simulink model "util_gravity_gradient_hrn"  (R2014b)
settings: Solver=VariableStepDiscrete  StartTime=0.0  StopTime=10.0  RelTol=1e-3
undefined symbols (not defined in the file or in its folder): csu_srp_solar_radiation_model_lib, gravity_gradient_torque, grv_mu_moon, I_sc, pos_m2sc_I, pos_sc2moon_body, q_body_from_mci
libraries: util_common_lib x9, util_info_lib x4, util_quat_lib x2
settings Model: Creator=Bryan Chan  LastModifiedBy=mstewart
settings DebuggingCC: UnderspecifiedInitializationDetection=Classic  MergeDetectMultiDrivingBlocksExec=none  SolverPrmCheckMsg=none  StateNameClashWarn=warning

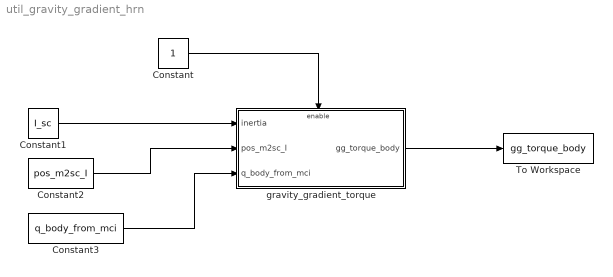
== system util_gravity_gradient_hrn ==
  Constant : Constant
  Constant1 : Constant  Value=I_sc
  Constant2 : Constant  Value=pos_m2sc_I
  Constant3 : Constant  Value=q_body_from_mci
  To Workspace : ToWorkspace  VariableName=gg_torque_body  SaveFormat=Timeseries  SampleTime=-1
  gravity_gradient_torque : Subsystem  AncestorBlock=csu_srp_solar_radiation_model_lib/gravity_gradient_torque
  wires:
  Constant/1 -> gravity_gradient_torque/Enable
  Constant1/1 -> gravity_gradient_torque/1(inertia)
  gravity_gradient_torque/1(gg_torque_body) -> To Workspace/1
  Constant2/1 -> gravity_gradient_torque/2(pos_m2sc_I)
  Constant3/1 -> gravity_gradient_torque/3(q_body_from_mci)

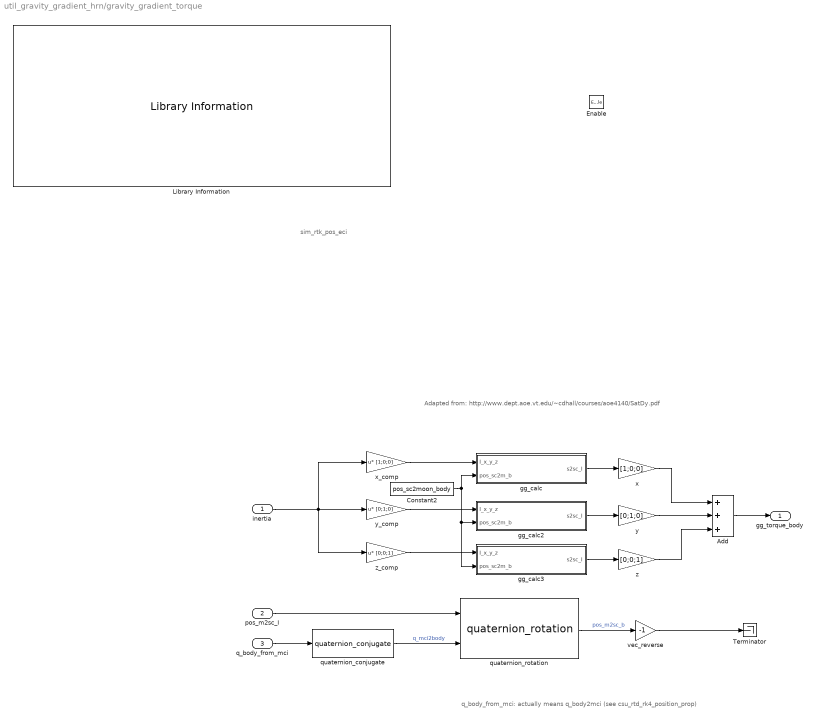
== system util_gravity_gradient_hrn/gravity_gradient_torque ==
  note: sim_rtk_pos_eci
  note: Adapted from: http://www.dept.aoe.vt.edu/~cdhall/courses/aoe4140/SatDy.pdf
  note: q_body_from_mci: actually means q_body2mci (see csu_rtd_rk4_position_prop)
  inertia : Inport
  pos_m2sc_I : Inport  Port=2
  q_body_from_mci : Inport  Port=3
  Enable : EnablePort
  Add : Sum  Inputs=+++
  Constant2 : Constant  Value=pos_sc2moon_body
  Library Information : util_info_lib/Library Information  owner='NONE'
  Terminator : Terminator
  gg_calc : Subsystem
  gg_calc2 : Subsystem
  gg_calc3 : Subsystem
  quaternion_conjugate : util_quat_lib/quaternion_conjugate  SystemSampleTime=-1
  quaternion_rotation : util_quat_lib/quaternion_rotation  SystemSampleTime=-1
  vec_reverse : Gain  Gain=-1
  x : Gain  Gain=[1;0;0]
  x_comp : Gain  Gain=[1;0;0]  Multiplication=Matrix(u*K)
  y : Gain  Gain=[0;1;0]
  y_comp : Gain  Gain=[0;1;0]  Multiplication=Matrix(u*K)
  z : Gain  Gain=[0;0;1]
  z_comp : Gain  Gain=[0;0;1]  Multiplication=Matrix(u*K)
  gg_torque_body : Outport
  wires:
  gg_calc3/1(s2sc_I) -> z/1
  gg_calc2/1(s2sc_I) -> y/1
  gg_calc/1(s2sc_I) -> x/1
  Constant2/1 -> gg_calc/2(pos_sc2m_b), gg_calc3/2(pos_sc2m_b), gg_calc2/2(pos_sc2m_b)
  z_comp/1 -> gg_calc3/1(I_x_y_z)
  y_comp/1 -> gg_calc2/1(I_x_y_z)
  x_comp/1 -> gg_calc/1(I_x_y_z)
  Add/1 -> gg_torque_body/1
  inertia/1 -> y_comp/1, z_comp/1, x_comp/1
  vec_reverse/1 -> Terminator/1
  quaternion_rotation/1 -> vec_reverse/1  "pos_m2sc_b"
  quaternion_conjugate/1 -> quaternion_rotation/2  "q_mci2body"
  q_body_from_mci/1 -> quaternion_conjugate/1
  pos_m2sc_I/1 -> quaternion_rotation/1
  x/1 -> Add/1
  y/1 -> Add/2
  z/1 -> Add/3

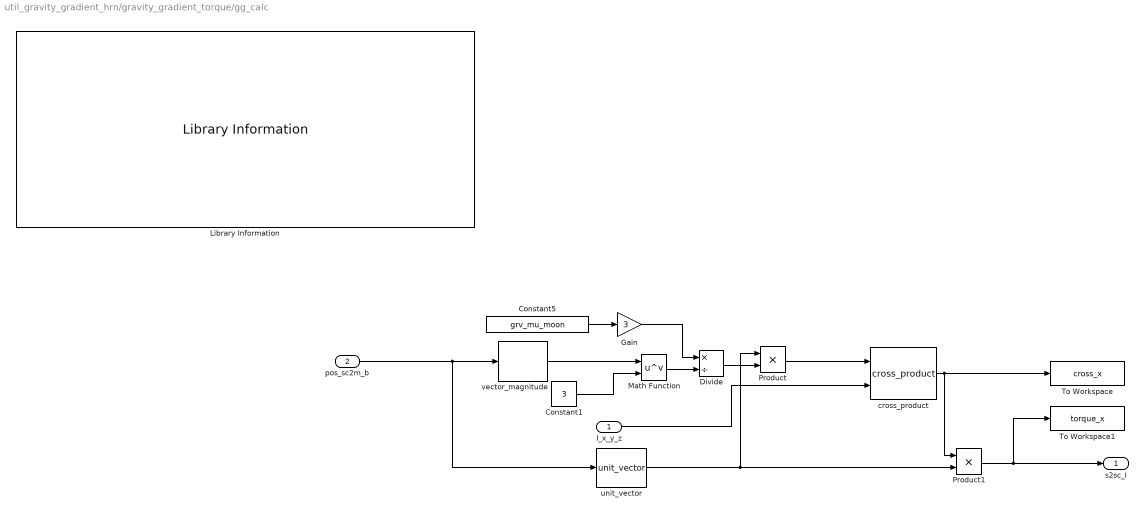
== system util_gravity_gradient_hrn/gravity_gradient_torque/gg_calc ==
  I_x_y_z : Inport
  pos_sc2m_b : Inport  Port=2
  Constant1 : Constant  Value=3
  Constant5 : Constant  Value=grv_mu_moon
  Divide : Product  Inputs=*/
  Gain : Gain  Gain=3
  Library Information : util_info_lib/Library Information  owner='NONE'
  Math Function : Math  Operator=pow  SaturateOnIntegerOverflow=on
  Product : Product
  Product1 : Product
  To Workspace : ToWorkspace  VariableName=cross_x  SaveFormat=Timeseries  SampleTime=-1
  To Workspace1 : ToWorkspace  VariableName=torque_x  SaveFormat=Timeseries  SampleTime=-1
  cross_product : util_common_lib/cross_product  SystemSampleTime=-1
  unit_vector : util_common_lib/unit_vector  SystemSampleTime=-1
  vector_magnitude : util_common_lib/vector_magnitude  SystemSampleTime=-1
  s2sc_I : Outport
  wires:
  pos_sc2m_b/1 -> vector_magnitude/1, unit_vector/1
  unit_vector/1 -> Product1/2, Product/1
  Math Function/1 -> Divide/2
  Gain/1 -> Divide/1
  Constant5/1 -> Gain/1
  Constant1/1 -> Math Function/2
  vector_magnitude/1 -> Math Function/1
  I_x_y_z/1 -> cross_product/2
  cross_product/1 -> Product1/1, To Workspace/1
  Divide/1 -> Product/2
  Product/1 -> cross_product/1
  Product1/1 -> To Workspace1/1, s2sc_I/1

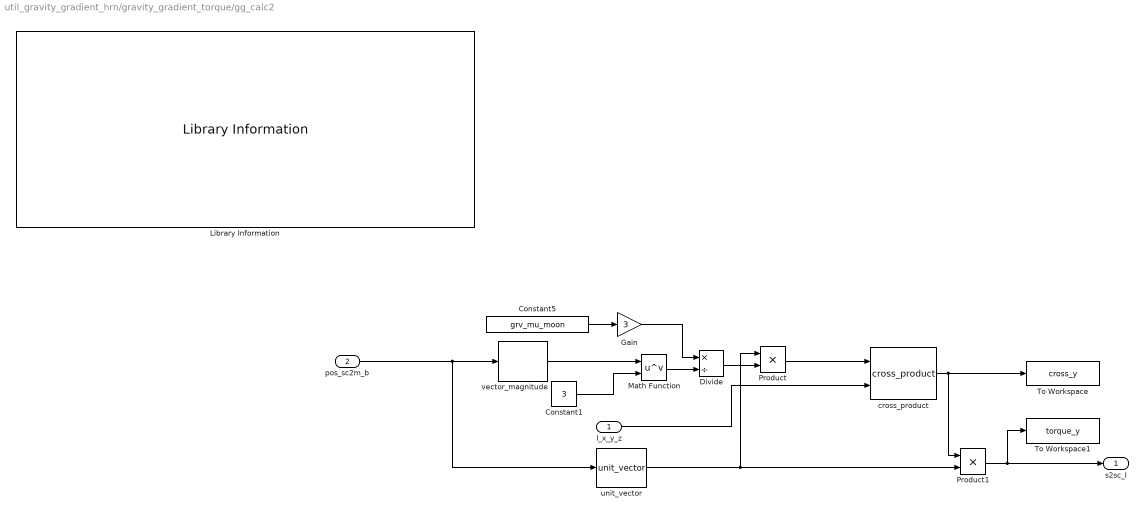
== system util_gravity_gradient_hrn/gravity_gradient_torque/gg_calc2 ==
  I_x_y_z : Inport
  pos_sc2m_b : Inport  Port=2
  Constant1 : Constant  Value=3
  Constant5 : Constant  Value=grv_mu_moon
  Divide : Product  Inputs=*/
  Gain : Gain  Gain=3
  Library Information : util_info_lib/Library Information  owner='NONE'
  Math Function : Math  Operator=pow  SaturateOnIntegerOverflow=on
  Product : Product
  Product1 : Product
  To Workspace : ToWorkspace  VariableName=cross_y  SaveFormat=Timeseries  SampleTime=-1
  To Workspace1 : ToWorkspace  VariableName=torque_y  SaveFormat=Timeseries  SampleTime=-1
  cross_product : util_common_lib/cross_product  SystemSampleTime=-1
  unit_vector : util_common_lib/unit_vector  SystemSampleTime=-1
  vector_magnitude : util_common_lib/vector_magnitude  SystemSampleTime=-1
  s2sc_I : Outport
  wires:
  Product1/1 -> To Workspace1/1, s2sc_I/1
  Product/1 -> cross_product/1
  Divide/1 -> Product/2
  cross_product/1 -> To Workspace/1, Product1/1
  I_x_y_z/1 -> cross_product/2
  vector_magnitude/1 -> Math Function/1
  Constant1/1 -> Math Function/2
  Constant5/1 -> Gain/1
  Gain/1 -> Divide/1
  Math Function/1 -> Divide/2
  unit_vector/1 -> Product1/2, Product/1
  pos_sc2m_b/1 -> unit_vector/1, vector_magnitude/1

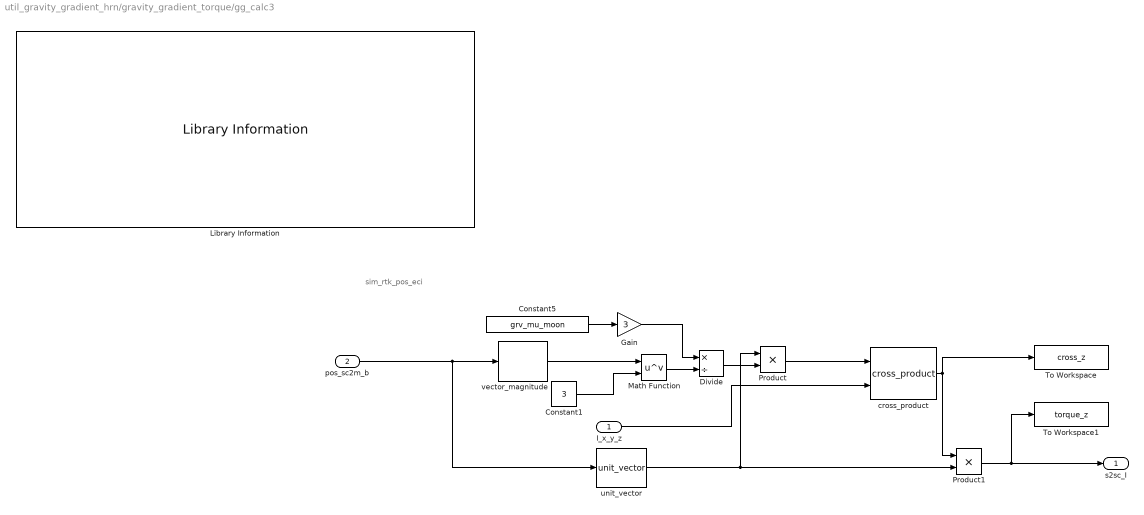
== system util_gravity_gradient_hrn/gravity_gradient_torque/gg_calc3 ==
  note: sim_rtk_pos_eci
  I_x_y_z : Inport
  pos_sc2m_b : Inport  Port=2
  Constant1 : Constant  Value=3
  Constant5 : Constant  Value=grv_mu_moon
  Divide : Product  Inputs=*/
  Gain : Gain  Gain=3
  Library Information : util_info_lib/Library Information  owner='NONE'
  Math Function : Math  Operator=pow  SaturateOnIntegerOverflow=on
  Product : Product
  Product1 : Product
  To Workspace : ToWorkspace  VariableName=cross_z  SaveFormat=Timeseries  SampleTime=-1
  To Workspace1 : ToWorkspace  VariableName=torque_z  SaveFormat=Timeseries  SampleTime=-1
  cross_product : util_common_lib/cross_product  SystemSampleTime=-1
  unit_vector : util_common_lib/unit_vector  SystemSampleTime=-1
  vector_magnitude : util_common_lib/vector_magnitude  SystemSampleTime=-1
  s2sc_I : Outport
  wires:
  pos_sc2m_b/1 -> vector_magnitude/1, unit_vector/1
  unit_vector/1 -> Product1/2, Product/1
  Math Function/1 -> Divide/2
  Gain/1 -> Divide/1
  Constant5/1 -> Gain/1
  Constant1/1 -> Math Function/2
  vector_magnitude/1 -> Math Function/1
  I_x_y_z/1 -> cross_product/2
  cross_product/1 -> Product1/1, To Workspace/1
  Divide/1 -> Product/2
  Product/1 -> cross_product/1
  Product1/1 -> To Workspace1/1, s2sc_I/1
